simulink model "test_breathing"  (R2026a)
settings: Solver=ode23t  StopTime=20  MaxStep=0.005
libraries: scuba_lib x8, nesl_utility x7
settings Model: Creator=grouleau  LastModifiedBy=grouleau

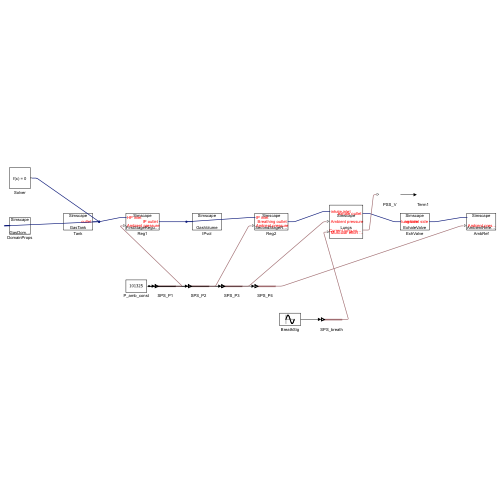
[thumbnail: Simulink's stored preview of the top-level diagram]
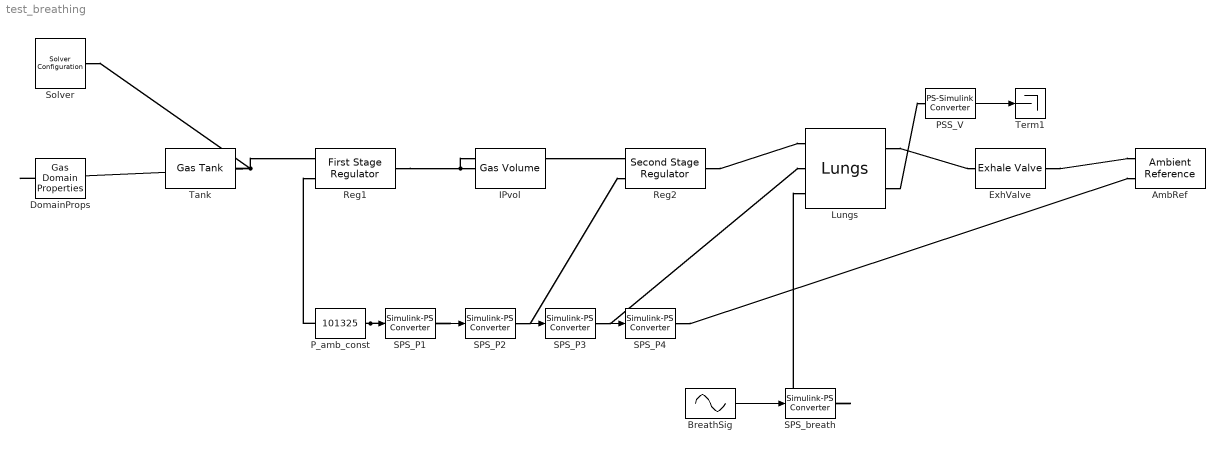
== system test_breathing ==
  AmbRef : scuba_lib/gas/elements/Ambient Reference  n_dot_in_specify=off  n_dot_in_priority=None  n_dot_in=0 mol/s  n_dot_in_nominal_specify=off  n_dot_in_nominal_value=1  n_dot_in_nominal_unit=mol/s
  BreathSig : Sin  Amplitude=200  Frequency=2*pi*0.25  SampleTime=0
  DomainProps : scuba_lib/gas/elements/Gas Domain Properties  R_gas=8.314 J/(K*mol)  T=293.15 K  n_dot_thru_specify=off  n_dot_thru_priority=None  n_dot_thru=0 mol/s  n_dot_thru_nominal_specify=off  n_dot_thru_nominal_value=1  n_dot_thru_nominal_unit=mol/s
  ExhValve : scuba_lib/gas/elements/Exhale Valve  P_crack=50 Pa  R_open=9000 Pa*s/mol  n_dot_specify=off  n_dot_priority=None  n_dot=0 mol/s  n_dot_nominal_specify=off  n_dot_nominal_value=1  n_dot_nominal_unit=mol/s
  IPvol : scuba_lib/gas/elements/Gas Volume  V=1e-4 m^3  n_init=0.04518 mol  n_dot_in_specify=off  n_dot_in_priority=None  n_dot_in=0 mol/s  n_dot_in_nominal_specify=off  n_dot_in_nominal_value=1  n_dot_in_nominal_unit=mol/s
  Lungs : scuba_lib/gas/elements/Lungs  n_init=0.0624 mol  n_dot_in_specify=off  n_dot_in_priority=None  n_dot_in=0 mol/s  n_dot_in_nominal_specify=off  n_dot_in_nominal_value=1  n_dot_in_nominal_unit=mol/s  n_dot_out_specify=off  n_dot_out_priority=None  n_dot_out=0 mol/s  n_dot_out_nominal_specify=off  n_dot_out_nominal_value=1  n_dot_out_nominal_unit=mol/s
  PSS_V : nesl_utility/PS-Simulink Converter  PhysicalDomain=network_engine_domain  SubClassName=ps_output  LeftPortType=input  RightPortType=output  PseudoPeriodic=off  Frequencies=[]  VectorFormat=inherit  Unit=m^3  AffineConversion=off
  P_amb_const : Constant  Value=101325
  Reg1 : scuba_lib/gas/elements/First Stage Regulator  IP_offset=10e5 Pa  R_open=1e3 Pa*s/mol  n_dot_specify=off  n_dot_priority=None  n_dot=0 mol/s  n_dot_nominal_specify=off  n_dot_nominal_value=1  n_dot_nominal_unit=mol/s
  Reg2 : scuba_lib/gas/elements/Second Stage Regulator  P_crack=100 Pa  R_open=6000 Pa*s/mol  n_dot_specify=off  n_dot_priority=None  n_dot=0 mol/s  n_dot_nominal_specify=off  n_dot_nominal_value=1  n_dot_nominal_unit=mol/s
  SPS_P{1..4} (4 alike) : nesl_utility/Simulink-PS Converter  PhysicalDomain=network_engine_domain  SubClassName=ps_input  LeftPortType=input  RightPortType=output  PseudoPeriodic=off  Frequencies=[]  NoiseDistribution=none  NoiseParameters=[]  Unit=Pa  AffineConversion=off  FilteringAndDerivatives=provide  SimscapeFilterOrder=1  InputFilterTimeConstant=0.001  UdotUserProvided=0
  SPS_breath : nesl_utility/Simulink-PS Converter  PhysicalDomain=network_engine_domain  SubClassName=ps_input  LeftPortType=input  RightPortType=output  PseudoPeriodic=off  Frequencies=[]  NoiseDistribution=none  NoiseParameters=[]  Unit=Pa  AffineConversion=off  FilteringAndDerivatives=provide  SimscapeFilterOrder=1  InputFilterTimeConstant=0.001  UdotUserProvided=0
  Solver : nesl_utility/Solver Configuration  PhysicalDomain=network_engine_domain  SubClassName=solver  LeftPortType=input  RightPortType=generic  Tones=[]  Harmonics=[]  SimulateNoise=off  Profile=off  UseLocalSampling=off  EnableSwitchedLinearOptims=on  FrequencyDomain=off  UseCCode=off  RelTol=0.001  AbsTol=0.001  MinStep=1e-09  ToWorkspace=off  RevertToSquareIcSolve=off  NumHomotopyIterations=100  PhasorMode=off  PhasorModeNumHarmonics=1  ConsistencySolver=NEWTON_XTOL_AFTER_FTOL  CanonicalOrdering=CANONICAL  OptimizeIntermediates=OPTIMIZED  IndexReductionMethod=DerivativeReplacement  DoDC=off  ResidualTolerance=1e-09  ConsistencyTolSource=GLOBAL  ConsistencyAbsTol=0.001  ConsistencyRelTol=0.001  ConsistencyTolFactor=0.001  UseLocalSolver=off  LocalSolverChoice=NE_BACKWARD_EULER_ADVANCER  ResolveIndetEquations=on  FunctionEvalNumThread=1  LocalSolverSampleTime=0.001  DoFixedCost=off  MaxNonlinIter=3  MaxModeIter=2  ComputeImpulses=off  ImpulseIterations=2  LinearAlgebra=auto  LinearAlgebraNumThread=0  EquationFormulation=NE_TIME_EF  DelaysMemoryBudget=1024  AutomaticFiltering=on  FilteringTimeConstant=0.001  PartitionStorageMethod=AS_NEEDED  PartitionMemoryBudget=1024  PartitionMethod=ROBUST  MultibodyUseLocalSolver=off  MultibodyLocalSolverChoice=ODE1  MultibodyLocalSolverSampleTime=0.001
  Tank : scuba_lib/gas/elements/Gas Tank  V_tank=0.012 m^3  n_init=98.47 mol  n_dot_out_specify=off  n_dot_out_priority=None  n_dot_out=0 mol/s  n_dot_out_nominal_specify=off  n_dot_out_nominal_value=1  n_dot_out_nominal_unit=mol/s
  Term1 : Terminator
  wires:
  P_amb_const/1 -> SPS_P1/1, SPS_P2/1, SPS_P3/1, SPS_P4/1
  BreathSig/1 -> SPS_breath/1
  PSS_V/1 -> Term1/1
  connections:
  DomainProps/LConn1 -- Reg1/LConn1 -- Tank/RConn1 -- Solver/RConn1
  IPvol/LConn1 -- Reg1/RConn1 -- Reg2/LConn1
  Reg2/RConn1 -- Lungs/LConn1
  Lungs/RConn1 -- ExhValve/LConn1
  ExhValve/RConn1 -- AmbRef/LConn1
  SPS_P1/RConn1 -- Reg1/LConn2
  SPS_P2/RConn1 -- Reg2/LConn2
  SPS_P3/RConn1 -- Lungs/LConn2
  SPS_P4/RConn1 -- AmbRef/LConn2
  SPS_breath/RConn1 -- Lungs/LConn3
  Lungs/RConn2 -- PSS_V/LConn1
